simulink library "ServoTrainer"  (Simulink 4.00)

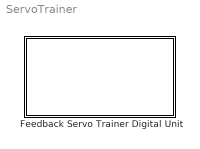
== system ServoTrainer ==
  Feedback Servo Trainer Digital Unit : Subsystem
      settings: RTWFcnNameOpts=Auto  RTWFileNameOpts=Auto
      mask Type: Feedback Servo Trainer Digital Unit
      mask Display: disp ('Feedback 33-003 \n\n Digital Servo Fundementals ')

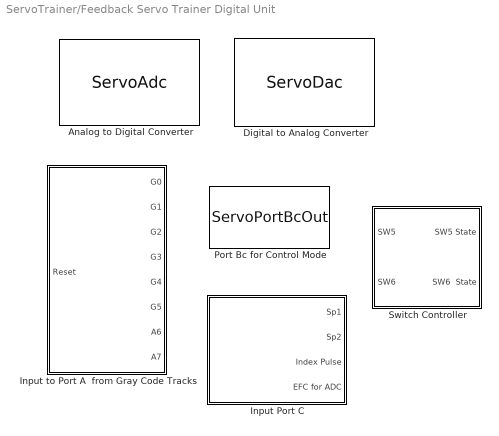
== system ServoTrainer/Feedback Servo Trainer Digital Unit ==
  Analog to Digital Converter : S-Function  FunctionName=ServoAdc  Parameters=inType,stime, hwAccess  PortCounts=[]  SFunctionModules=''  mask(Analog to Digital Converter){inType=RawData (-127 to +127), stime=0.01, hwAccess=on}
      mask prompts: inType "Input Type"; stime "Sampling Time (sec.)"; hwAccess "Access Hardware"
      mask help:
      | Analog Input Unit for Feedback DU154B
      | Digital Unit 33-003
      | Feeback Instruments
      mask Help:
      | Reads and converts the voltage applied to ADC input on the Digital Unit.
      | Read operation is done either in Rawdata (+/- 127) format or directly in voltage format
      mask StyleString: popup(RawData (-127 to +127)| Volt   (+/- 11V range)),edit,checkbox
      mask Display: disp('Feedback Servo Trainer\n Digital Unit 33-003\n\n ADC')
  Digital to Analog Converter : S-Function  FunctionName=ServoDac  Parameters=outType,stime, hwAccess  PortCounts=[]  SFunctionModules=''  mask(Analog Output Module){outType=RawData (-127 to +127), stime=0.01, hwAccess=on}
      mask prompts: outType "Output Type :"; stime "Sampling Time (sec.)"; hwAccess "Access Hardware"
      mask help:
      | Analog Output Unit for Feedback DU154B
      | Digital Unit 33-003
      | Feeback Instruments
      mask Help:
      | Applies the corresponding voltage to the Servo Trainers DAC
      | output type can be selected to be either in RawData type or directly in volts
      mask StyleString: popup(RawData (-127 to +127)| Volt   (+/- 11V range)),edit,checkbox
      mask Display: disp('Feedback Servo Trainer\n Digital Unit 33-003\n\n DAC')
  Input Port C : Subsystem  mask(Read the Inputs from portC directly){stime=0.01, hwAccess=on}
      mask prompts: stime "Sample Time (sec.)"; hwAccess "Access Hardware"
      settings: RTWFcnNameOpts=Auto  RTWFileNameOpts=Auto
  Input to Port A  from Gray Code Tracks : Subsystem  mask(Read Gray Code and Speed Tracks){stime=0.01, hwAccess=on}
      mask prompts: stime "Sample Time (sec.)"; hwAccess "Hardware Access"
      mask help:
      | Read the inputs from the Gray Code tracks (A0-A5)
      | and Speed/Increment tracks (A6-A7)
      settings: RTWFcnNameOpts=Auto  RTWFileNameOpts=Auto
      mask Help: no help is available for this block
  Port Bc for Control Mode : S-Function  FunctionName=ServoPortBcOut  Parameters=stime, hwAccess  PortCounts=[]  SFunctionModules=''  mask(Port Bc for Direct access to Control Signals){stime=0.01, hwAccess=on}
      mask prompts: stime "Sample Time (sec.)"; hwAccess "Access Hardware"
      mask help:
      | To directly access the Bc control register
      | For Advanced users only !
      mask Help:
      | Will directly apply the integer input to the Bc control output
      | This module is for advenced users only .
      | using this module with other Servo Trainer modules may corrupt inputs !
      mask Display: disp('Feedback Servo Trainer\n Digital Unit 33-003\n\nPort Bc')
  Switch Controller : Subsystem  mask(Switch Controller){onWhen=1, stime=0.01, hwAccess=on}
      mask prompts: onWhen "Thresh Hold"; stime "Sample Time (sec.)"; hwAccess "Hardware Access"
      mask help:
      | Controls the SW5 and SW6 switches on the Digital Unit
      | The ouptut can be used to see the state of the switches
      settings: RTWFcnNameOpts=Auto  RTWFileNameOpts=Auto
      mask Help: The Switches will be on when the input to the Swiches are bigger than or equal to the "Thresh Hold" variable

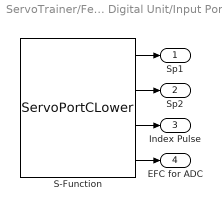
== system ServoTrainer/Feedback Servo Trainer Digital Unit/Input Port C ==
  S-Function : S-Function  FunctionName=ServoPortCLower  Parameters=stime, hwAccess  PortCounts=[]  SFunctionModules=''
  Sp1 : Outport  Port=1
  Sp2 : Outport  Port=2
  Index Pulse : Outport  Port=3
  "EFC for ADC  " : Outport  Port=4
  wires:
  S-Function/1 -> Sp1/1
  S-Function/2 -> Sp2/1
  S-Function/3 -> Index Pulse/1
  S-Function/4 -> "EFC for ADC  "/1

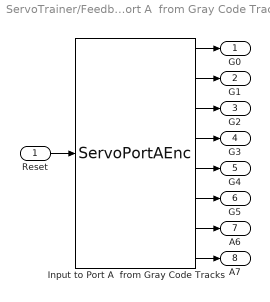
== system ServoTrainer/Feedback Servo Trainer Digital Unit/Input to Port A  from Gray Code Tracks ==
  Reset : Inport  Port=1
  Input to Port A  from Gray Code Tracks : S-Function  FunctionName=ServoPortAEnc  Parameters=stime,hwAccess  PortCounts=[]  SFunctionModules=''
  G0 : Outport  Port=1
  G1 : Outport  Port=2
  G2 : Outport  Port=3
  G3 : Outport  Port=4
  G4 : Outport  Port=5
  G5 : Outport  Port=6
  A6 : Outport  Port=7
  A7 : Outport  Port=8
  wires:
  Input to Port A  from Gray Code Tracks/1 -> G0/1
  Input to Port A  from Gray Code Tracks/2 -> G1/1
  Input to Port A  from Gray Code Tracks/3 -> G2/1
  Input to Port A  from Gray Code Tracks/4 -> G3/1
  Reset/1 -> Input to Port A  from Gray Code Tracks/1
  Input to Port A  from Gray Code Tracks/5 -> G4/1
  Input to Port A  from Gray Code Tracks/6 -> G5/1
  Input to Port A  from Gray Code Tracks/7 -> A6/1
  Input to Port A  from Gray Code Tracks/8 -> A7/1

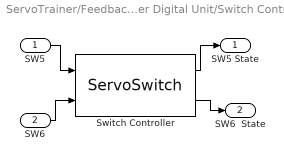
== system ServoTrainer/Feedback Servo Trainer Digital Unit/Switch Controller ==
  SW5 : Inport  Port=1
  SW6 : Inport  Port=2
  Switch Controller : S-Function  FunctionName=ServoSwitch  Parameters=onWhen,stime, hwAccess  PortCounts=[]  SFunctionModules=''
  SW5 State : Outport  Port=1
  SW6  State : Outport  Port=2
  wires:
  Switch Controller/1 -> SW5 State/1
  SW5/1 -> Switch Controller/1
  Switch Controller/2 -> SW6  State/1
  SW6/1 -> Switch Controller/2
